simulink library "models"  (Simulink 7.2)
settings: Solver=ode45  SolverMode=SingleTasking  StartTime=0.0  StopTime=10.0  RelTol=1e-3
undefined symbols (not defined in the file or in its folder): actuator_T2_lib, aero, Aero, aero_lib, aftfuel, aftfuel_pos, Am, atmos, b, bias, Bm, Cbar, cg_pos0, cg_shift_gear, constants, DamageModels, Ed_trim_IC, engl_ang, engl_pos, engr_ang, engr_pos, fwdfuel, fwdfuel_pos, GTM_T2, hd_trim_IC, in_tadapton_forced, Inertia0, Inertia_shift_gear, latlonh_IC, MACH_U_nom_IC, Nd_trim_IC, pqr_trim_IC, quat_trim_IC, ref_cg, S, SENSOR, SERVO, symmetric_aero_on, trac_params, use_wind_meas_sim, vehicle_params, w0, xm0
libraries: simulink_need_slupdate x56, models x11, aeroutilslib x6, utility_lib x5, GTM_aerolib x4, model_lib x4, Polyval_lib x3, simulink x2, enginelib x2, engine_T2_lib x1
(part 4 of 4)

== matlab function gtm-aero (for V0905)/Eng_GTM_T2/Engine Alignment ==
  data: T output double; Tl input double; hl input double; Tr input double; hr input double; TL output double; engl_ang parameter double; engr_ang parameter double; TR output double; H output double
function [T,TL,TR,H] = eng_angles(Tl,hl,Tr,hr,engl_ang,engr_ang)
% This block supports an embeddable subset of the MATLAB language.
% See the help menu for details. 

% Using the engine alignment angles (set in AC_params_T2.m), compute the 
% off-axis thrust and angular momentum terms.

TL = Tl*[cosd(engl_ang(2))*cosd(engl_ang(3));...
         -sind(engl_ang(3));...
         sind(engl_ang(2))*cosd(engl_ang(3))];
TR = Tr*[cosd(engr_ang(2))*cosd(engr_ang(3));...
         -sind(engr_ang(3));...
         sind(engr_ang(2))*cosd(engr_ang(3))];  
T = TL+TR;

H = hl*[cosd(engl_ang(2))*cosd(engl_ang(3));...
         -sind(engl_ang(3));...
         sind(engl_ang(2))*cosd(engl_ang(3))] + ...
         hr*[cosd(engr_ang(2))*cosd(engr_ang(3));...
         -sind(engr_ang(3));...
         sind(engr_ang(2))*cosd(engr_ang(3))];
